simulink model "controller_arduino"  (R2023b)
settings: Solver=FixedStepAuto  StartTime=0.0  StopTime=10.0  FixedStep=1/100  RelTol=1e-3
values from neighbouring files (symbols this model uses):
  MAX_TORQUE = 80    [init_fn.m]
  MAX_TORQUE_REVERSE = 40    [init_fn.m]
undefined symbols (not defined in the file or in its folder): MAX_SPEED_BACKWARD
libraries: arduinolib x17
settings Model: ExtModeTrigDuration=2  Creator=DAUIN-Win10  LastModifiedBy=Utilisateur
settings OptimizationCC: EnhancedBackFolding=on  PassReuseOutputArgsAs=Individual arguments  ZeroExternalMemoryAtStartup=off  ZeroInternalMemoryAtStartup=off  MaxStackSize=64  OptimizeBlockOrder=speed  DifferentSizesBufferReuse=on  OptimizationCustomize=off  EfficientTunableParamExpr=on
settings DebuggingCC: ParameterTunabilityLossMsg=error  UnconnectedInputMsg=warning  UnconnectedOutputMsg=warning  UnconnectedLineMsg=warning  UnderSpecifiedDimensionMsg=error
settings HardwareCC: ProdBitPerInt=16  ProdBitPerPointer=16  ProdBitPerSizeT=16  ProdBitPerPtrDiffT=16  ProdLargestAtomicFloat=None  ProdWordSize=8  ProdHWDeviceType=Atmel->AVR
settings ModelReferenceCC: EnableRefExpFcnMdlSchedulingChecks=on
settings SFSimCC: MATLABDynamicMemAlloc=off
settings RTWCC: Description=Embedded Coder  SystemTargetFile=ert.tlc  HardwareBoard=Arduino Uno  TemplateMakefile=ert_default_tmf  Toolchain=Arduino AVR  DLArmComputeVersion=19.05
settings CodeAppCC: ForceParamTrailComments=on  IgnoreCustomStorageClasses=off  OperatorAnnotations=on  SimulinkDataObjDesc=on  SFDataObjDesc=on  InsertBlockDesc=on
settings ERTTargetCC: SupportContinuousTime=on  SupportVariableSizeSignals=on  ExtModeTransport=3  ExtModeStaticAlloc=on  ExtModeAutomaticAllocSize=off  ExtModeStaticAllocSize=250  ExtModeMexFile=ext_xcp  ExtModeIntrfLevel=Level2 - Open

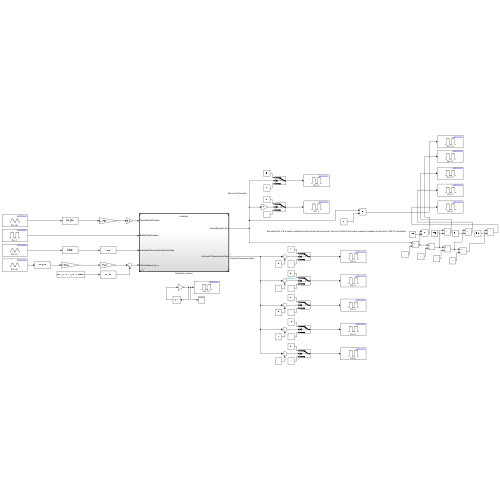
[thumbnail: Simulink's stored preview of the top-level diagram]
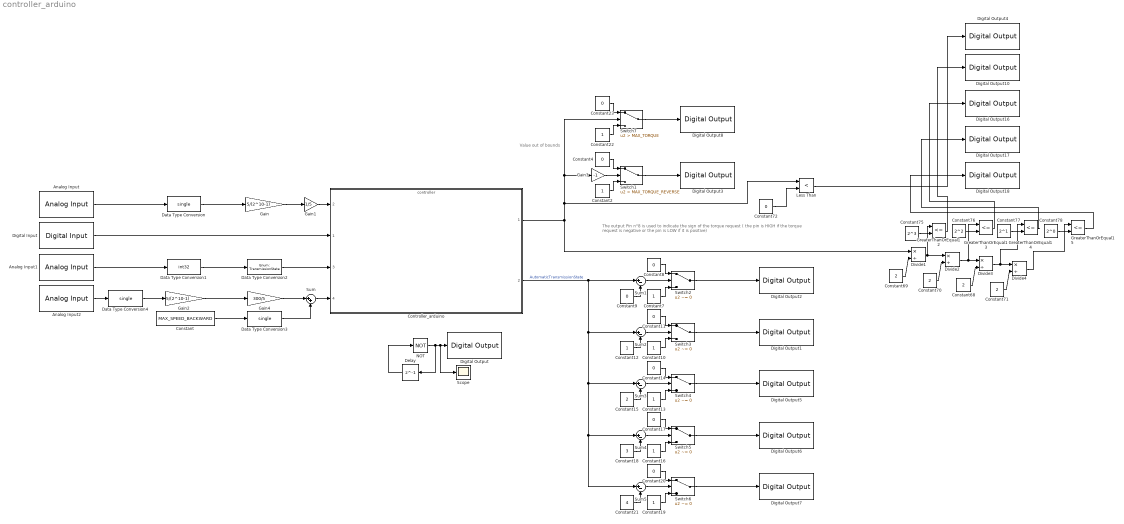
== system controller_arduino ==
  note: The output Pin n°8 is used to indicate the sign of the torque request ( the pin is HIGH if the torque request is negative or the pin is LOW if it is positive)
  note: Value out of bounds
  Analog Input : arduinolib/Analog Input  pinNumber=0  ReadResultsOnly=off  ConversionTriggerSource=Software  ExternalTriggerType=uint32( 0 )  OutputDataType=uint16  EnableConversionCompleteNotify=off  EnableOuputStatus=off  SampleTime=-1  blockPlatform=arduino
  Analog Input1 : arduinolib/Analog Input  pinNumber=1  ReadResultsOnly=off  ConversionTriggerSource=Software  ExternalTriggerType=uint32( 0 )  OutputDataType=uint16  EnableConversionCompleteNotify=off  EnableOuputStatus=off  SampleTime=-1  blockPlatform=arduino
  Analog Input2 : arduinolib/Analog Input  pinNumber=2  ReadResultsOnly=off  ConversionTriggerSource=Software  ExternalTriggerType=uint32( 0 )  OutputDataType=uint16  EnableConversionCompleteNotify=off  EnableOuputStatus=off  SampleTime=-1  blockPlatform=arduino
  Constant : Constant  Value=MAX_SPEED_BACKWARD
  Constant{2,7,10,12..13,16,19,22} (8 alike) : Constant
  Constant{4,8..9,11,14,17,20,23,72} (9 alike) : Constant  Value=0
  Constant{15,68..71} (5 alike) : Constant  Value=2
  Constant18 : Constant  Value=3
  Constant21 : Constant  Value=4
  Constant75 : Constant  Value=2^3
  Constant76 : Constant  Value=2^2
  Constant77 : Constant  Value=2^1
  Constant78 : Constant  Value=2^0
  Controller_arduino : ModelReference  ModelNameDialog=controller  SimulationMode=Normal  ModelReferenceVersion=5.57
      settings: PortSchema="{\"entries\":[{\"content\":{\"sides\":[{\"content\":{\"connectorIds\":[\"In2\",\"In1\",\"In3\",\"In4\"]},\"type\":\"ConnectorPlacement.EquallySpacedRectSide\",\"uuid\":\"5e260b81-e1ce-497c-8572-ac5c2182ee27\"},{\"content\":{\"connectorIds\":[\"Out1\",\"Out2\"],\"side\":\"RIGHT\"},\"type\":\"ConnectorPlacement.EquallySpacedRectSide\",\"uuid\":\"4325f63c-e453-4c79-ab01-1476da99aa25\"},{\"content\":{\"connectorIds\":[],\"side\":\"TOP\"},\"type\":\"ConnectorPlacement.EquallySpacedRectSide\",\"uuid\":\"dba88bac-0f95-4a98-ba3b-c40df5616f56\"}]},\"type\":\"ConnectorPlacement.EquallySpacedConnector\",\"uuid\":\"6943e10d-f3b0-4fd8-a142-b6b49e651f90\"}],\"packageUris\":[\"http://schema.mathworks.com/mf0/Connector/R2020b\"],\"version\":\"1.0\"}"
  Data Type Conversion : DataTypeConversion  OutDataTypeStr=single  SaturateOnIntegerOverflow=off  RndMeth=Floor
  Data Type Conversion1 : DataTypeConversion  OutDataTypeStr=int32  SaturateOnIntegerOverflow=off  RndMeth=Floor
  Data Type Conversion2 : DataTypeConversion  OutDataTypeStr=Enum: TransmissionState  SaturateOnIntegerOverflow=off  RndMeth=Floor
  Data Type Conversion3 : DataTypeConversion  OutDataTypeStr=single  SaturateOnIntegerOverflow=off  RndMeth=Floor
  Data Type Conversion4 : DataTypeConversion  OutDataTypeStr=single  SaturateOnIntegerOverflow=off  RndMeth=Floor
  Delay : Delay  DelayLength=1
  Digital Input : arduinolib/Digital Input  pinNumber=7  mode=Default  Direction=input  SampleTime=-1  blockPlatform=arduino
  Digital Output : arduinolib/Digital Output  pinNumber=13  Direction=output  blockPlatform=arduino
  Digital Output1 : arduinolib/Digital Output  pinNumber=3  Direction=output  blockPlatform=arduino
  Digital Output10 : arduinolib/Digital Output  pinNumber=11  Direction=output  blockPlatform=arduino
  Digital Output16 : arduinolib/Digital Output  pinNumber=10  Direction=output  blockPlatform=arduino
  Digital Output17 : arduinolib/Digital Output  pinNumber=9  Direction=output  blockPlatform=arduino
  Digital Output18 : arduinolib/Digital Output  pinNumber=8  Direction=output  blockPlatform=arduino
  Digital Output2 : arduinolib/Digital Output  pinNumber=2  Direction=output  blockPlatform=arduino
  Digital Output3 : arduinolib/Digital Output  pinNumber=1  Direction=output  blockPlatform=arduino
  Digital Output4 : arduinolib/Digital Output  pinNumber=12  Direction=output  blockPlatform=arduino
  Digital Output5 : arduinolib/Digital Output  pinNumber=4  Direction=output  blockPlatform=arduino
  Digital Output6 : arduinolib/Digital Output  pinNumber=5  Direction=output  blockPlatform=arduino
  Digital Output7 : arduinolib/Digital Output  pinNumber=6  Direction=output  blockPlatform=arduino
  Digital Output8 : arduinolib/Digital Output  pinNumber=0  Direction=output  blockPlatform=arduino
  Divide{1..4} (4 alike) : Product  Inputs=*/
  Gain : Gain  Gain=5/(2^10-1)
  Gain1 : Gain  Gain=1/5
  Gain2 : Gain  Gain=5/(2^10-1)
  Gain3 : Gain  Gain=-1
  Gain4 : Gain  Gain=300/5
  GreaterThanOrEqual{12..15} (4 alike) : RelationalOperator  Operator=<=  OutDataTypeStr=boolean  RndMeth=Simplest  InputSameDT=off
  Less Than : RelationalOperator  Operator=<  OutDataTypeStr=boolean  RndMeth=Simplest  InputSameDT=off
  NOT : Logic  Operator=NOT  IconShape=distinctive  AllPortsSameDT=off  OutDataTypeStr=boolean
  Scope : Scope
  Sum : Sum  Inputs=|++
  Sum{1..5} (5 alike) : Sum  Inputs=|+-
  Switch1 : Switch  Criteria=u2 > Threshold  Threshold=MAX_TORQUE_REVERSE  SaturateOnIntegerOverflow=off  InputSameDT=off
  Switch{2..6} (5 alike) : Switch  Criteria=u2 ~= 0  Threshold=MAX_TORQUE_REVERSE  SaturateOnIntegerOverflow=off  InputSameDT=off
  Switch7 : Switch  Criteria=u2 > Threshold  Threshold=MAX_TORQUE  SaturateOnIntegerOverflow=off  InputSameDT=off
  wires:
  NOT/1 -> Delay/1, Scope/1, Digital Output/1
  Delay/1 -> NOT/1
  Analog Input/1 -> Data Type Conversion/1
  Analog Input2/1 -> Data Type Conversion4/1
  Data Type Conversion/1 -> Gain/1
  Gain/1 -> Gain1/1
  Gain1/1 -> Controller_arduino/2
  Data Type Conversion1/1 -> Data Type Conversion2/1
  Data Type Conversion2/1 -> Controller_arduino/3
  Data Type Conversion4/1 -> Gain2/1
  Gain2/1 -> Gain4/1
  Gain4/1 -> Sum/1
  Sum/1 -> Controller_arduino/4
  Constant/1 -> Data Type Conversion3/1
  Digital Input/1 -> Controller_arduino/1
  Data Type Conversion3/1 -> Sum/2
  Analog Input1/1 -> Data Type Conversion1/1
  Gain3/1 -> Switch1/2
  Constant2/1 -> Switch1/3
  Constant4/1 -> Switch1/1
  Switch1/1 -> Digital Output3/1
  Constant8/1 -> Switch2/1
  Constant7/1 -> Switch2/3
  Sum1/1 -> Switch2/2
  Constant9/1 -> Sum1/2
  Constant12/1 -> Sum2/2
  Sum2/1 -> Switch3/2
  Constant10/1 -> Switch3/3
  Constant11/1 -> Switch3/1
  Constant14/1 -> Switch4/1
  Constant13/1 -> Switch4/3
  Sum3/1 -> Switch4/2
  Constant15/1 -> Sum3/2
  Constant18/1 -> Sum4/2
  Sum4/1 -> Switch5/2
  Constant16/1 -> Switch5/3
  Constant17/1 -> Switch5/1
  Constant20/1 -> Switch6/1
  Constant19/1 -> Switch6/3
  Sum5/1 -> Switch6/2
  Constant21/1 -> Sum5/2
  Controller_arduino/2 -> Sum5/1, Sum4/1, Sum3/1, Sum2/1, Sum1/1  "AutomaticTransmissionState"
  Switch2/1 -> Digital Output2/1
  Switch3/1 -> Digital Output1/1
  Switch4/1 -> Digital Output5/1
  Switch6/1 -> Digital Output7/1
  Switch5/1 -> Digital Output6/1
  Switch7/1 -> Digital Output8/1
  Constant23/1 -> Switch7/1
  Constant22/1 -> Switch7/3
  Controller_arduino/1 -> Less Than/1, Switch7/2, Gain3/1, Divide1/1
  Constant69/1 -> Divide1/2
  Constant70/1 -> Divide2/2
  Constant68/1 -> Divide3/2
  Constant71/1 -> Divide4/2
  Divide1/1 -> GreaterThanOrEqual12/1, Divide2/1
  Divide2/1 -> GreaterThanOrEqual13/1, Divide3/1
  Divide3/1 -> GreaterThanOrEqual14/1, Divide4/1
  Divide4/1 -> GreaterThanOrEqual15/1
  Constant75/1 -> GreaterThanOrEqual12/2
  Constant76/1 -> GreaterThanOrEqual13/2
  Constant77/1 -> GreaterThanOrEqual14/2
  Constant78/1 -> GreaterThanOrEqual15/2
  GreaterThanOrEqual12/1 -> Digital Output10/1
  GreaterThanOrEqual13/1 -> Digital Output16/1
  GreaterThanOrEqual14/1 -> Digital Output17/1
  GreaterThanOrEqual15/1 -> Digital Output18/1
  Constant72/1 -> Less Than/2
  Less Than/1 -> Digital Output4/1
